simulink model "Teensy41_Cart_Pendulum_SysId"  (R2024b)
settings: Solver=FixedStepAuto  StartTime=0.0  StopTime=18  RelTol=1e-3  EnableMultiTasking=on
InitFcn:
  | run('Teensy41_system_init.m');
StopFcn:
  | run('Teensy41_to_save_data.m');
values from neighbouring files (symbols this model uses):
  Hz_den = Hz.denominator{1}    [Teensy41_system_init.m]
  Hz_num = Hz.numerator{1}    [Teensy41_system_init.m]
  ts = time(2)    [CartPend_SysId.m]    (also in Teensy41_system_init.m = 0.0025)
undefined symbols (not defined in the file or in its folder): dspblkCoreblockFVToolHelper, gcbh
libraries: arduinolib x9, simulink x2, simulink_extras x1
settings Model: SimulationMode=external  ExtModeTrigDuration=2  Creator=ricardoaguilera  LastModifiedBy=ricardoaguilera
settings SolverCC: AutoInsertRateTranBlk=on
settings OptimizationCC: EnhancedBackFolding=on  PassReuseOutputArgsAs=Individual arguments  ZeroExternalMemoryAtStartup=off  ZeroInternalMemoryAtStartup=off  MaxStackSize=64  OptimizeBlockOrder=speed  DifferentSizesBufferReuse=on  OptimizationCustomize=off  EfficientTunableParamExpr=on
settings DebuggingCC: ParameterTunabilityLossMsg=error
settings HardwareCC: ProdBitPerPointer=32  ProdBitPerSizeT=32  ProdBitPerPtrDiffT=32  ProdLargestAtomicInteger=Long  ProdLargestAtomicFloat=Double  ProdWordSize=32  ProdHWDeviceType=ARM Compatible->ARM Cortex
settings SFSimCC: MATLABDynamicMemAlloc=off
settings RTWCC: Description=Embedded Coder  SystemTargetFile=ert.tlc  HardwareBoard=Teensy 4.1 (Arduino Compatible)  TemplateMakefile=ert_default_tmf  Toolchain=Arduino ARM M7  BuildConfiguration=Faster Runs
settings CodeAppCC: ForceParamTrailComments=on  IgnoreCustomStorageClasses=off  OperatorAnnotations=on  SimulinkDataObjDesc=on  SFDataObjDesc=on  InsertBlockDesc=on
settings ERTTargetCC: SupportContinuousTime=on  SupportVariableSizeSignals=on  ExtModeTransport=3  ExtModeStaticAlloc=on  ExtModeAutomaticAllocSize=off  ExtModeStaticAllocSize=65536  ExtModeMexFile=ext_xcp  ExtModeIntrfLevel=Level2 - Open  InlinedParameterPlacement=Hierarchical

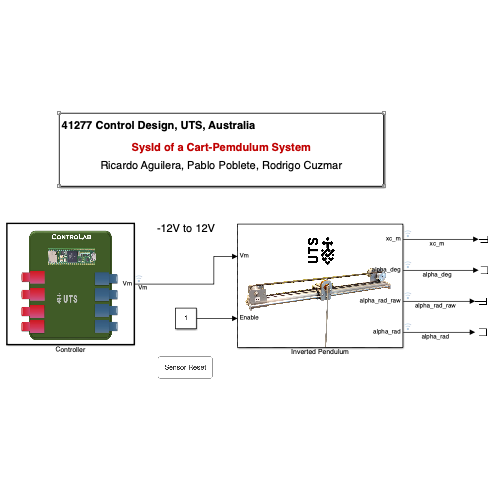
[thumbnail: Simulink's stored preview of the top-level diagram]
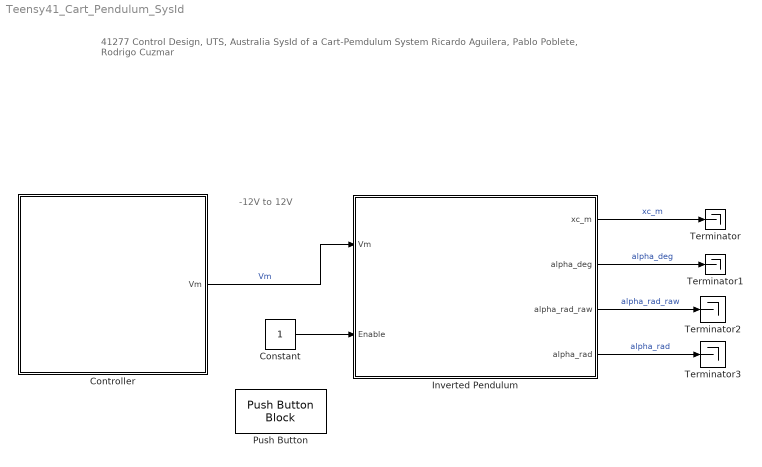
== system Teensy41_Cart_Pendulum_SysId ==
  note: 41277 Control Design, UTS, Australia
      |
      | SysId of a Cart-Pemdulum System
      |
      | Ricardo Aguilera, Pablo Poblete, Rodrigo Cuzmar
  note: -12V to 12V
  Constant : Constant
  Controller : Subsystem  TreatAsAtomicUnit=on
      mask Display: image('Board.png');
  Inverted Pendulum : Subsystem
      mask Display: image('bitmap.png');
  Push Button : PushButtonBlock  ButtonText=Sensor Reset  OffValue=0.000000
  Terminator{,1..3} (4 alike) : Terminator
  wires:
  Inverted Pendulum/1(xc_m) -> Terminator/1  "xc_m"
  Controller/1(Vm) -> Inverted Pendulum/1(Vm)  "Vm"
  Constant/1 -> Inverted Pendulum/2(Enable)
  Inverted Pendulum/4(alpha_rad) -> Terminator3/1  "alpha_rad"
  Inverted Pendulum/3(alpha_rad_raw) -> Terminator2/1  "alpha_rad_raw"
  Inverted Pendulum/2(alpha_deg) -> Terminator1/1  "alpha_deg"

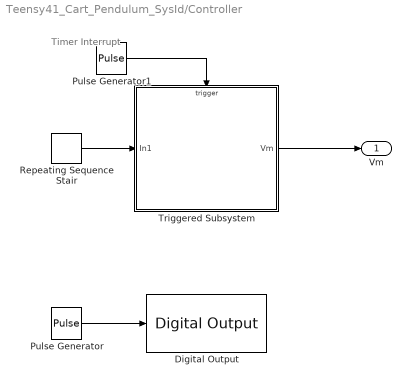
== system Teensy41_Cart_Pendulum_SysId/Controller ==
  note: Timer
      | Interrupt
  Digital Output : arduinolib/Digital Output  pinNumber=13  Direction=output  blockPlatform=arduino
      settings: SourceProductName=Common
  Pulse Generator : DiscretePulseGenerator  PulseType=Time based  Period=4  PulseWidth=50
  Pulse Generator1 : DiscretePulseGenerator  PulseType=Time based  Period=ts  PulseWidth=50
  Repeating Sequence Stair : simulink/Sources/Repeating Sequence Stair  OutValues=6*[0 1 0 0 0 0 0 0 0 -1 0 0 0 0 0 0 0].'  tsamp=1  OutMin=[]  OutMax=[]  OutDataTypeStr=double  OutputDataTypeScalingMode=double  OutDataType=fixdt(0,8)  ConRadixGroup=Best Precision: Vector-wise  OutScaling=2^-12
  Triggered Subsystem : Subsystem  TreatAsAtomicUnit=on
  Vm : Outport
  wires:
  Pulse Generator/1 -> Digital Output/1
  Triggered Subsystem/1(Vm) -> Vm/1
  Pulse Generator1/1 -> Triggered Subsystem/Trigger
  Repeating Sequence Stair/1 -> Triggered Subsystem/1(In1)

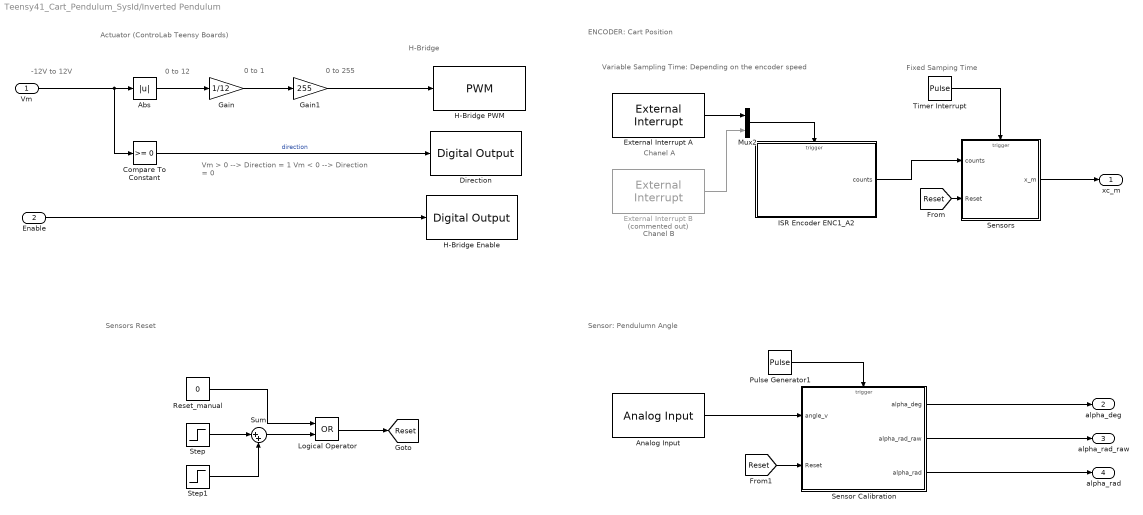
== system Teensy41_Cart_Pendulum_SysId/Inverted Pendulum ==
  note: Fixed Samping Time
  note: H-Bridge
  note: Variable Sampling Time: Depending on the encoder speed
  note: Chanel B
  note: 0 to 1
  note: Sensors Reset
  note: 0 to 12
  note: Chanel A
  note: ENCODER: Cart Position
  note: -12V to 12V
  note: 0 to 255
  note: Vm > 0 --> Direction = 1
      | Vm < 0 --> Direction = 0
  note: Sensor: Pendulumn Angle
  note: Actuator (ControLab Teensy Boards)
  Vm : Inport
  Enable : Inport  Port=2
  Abs : Abs  SaturateOnIntegerOverflow=off
  Analog Input : arduinolib/Analog Input  pinNumber=0  ReadResultsOnly=off  ConversionTriggerSource=Software  ExternalTriggerType=uint32( 0 )  OutputDataType=uint16  EnableConversionCompleteNotify=off  EnableOuputStatus=off  SampleTime=ts  blockPlatform=arduino
      settings: SourceProductName=Common
  Compare To Constant : simulink/Logic and Bit Operations/Compare To Constant  relop=>=  const=0  OutDataTypeStr=boolean
  Direction : arduinolib/Digital Output  pinNumber=8  Direction=output  blockPlatform=arduino
      settings: SourceProductName=Common
  "External Interrupt A " : arduinolib/External Interrupt  Pin=29  PullUp=off  Mode=CHANGE  InterruptSimulationInput=off
      settings: SourceProductName=Common
  External Interrupt B : arduinolib/External Interrupt  Commented=on  Pin=5  PullUp=off  Mode=CHANGE  InterruptSimulationInput=off
      settings: SourceProductName=Common
  Gain : Gain  Gain=1/12
  Gain1 : Gain  Gain=255
  H-Bridge Enable : arduinolib/Digital Output  pinNumber=9  Direction=output  blockPlatform=arduino
      settings: SourceProductName=Common
  H-Bridge PWM : arduinolib/PWM  pinNumber=3  frequencyType=Specify  desiredFrequency=10000  achievableFrequency=10000
      settings: SourceProductName=Common
  ISR Encoder ENC1_A2 : Subsystem  TreatAsAtomicUnit=on
  Logical Operator : Logic  Operator=OR  AllPortsSameDT=off  OutDataTypeStr=boolean
  Mux2 : Mux  Inputs=2
  Pulse Generator1 : DiscretePulseGenerator  PulseType=Time based  Period=ts  PulseWidth=50
  Reset_manual : Constant  Value=0  SampleTime=-1
  Sensor Calibration : Subsystem
  Sensors : Subsystem
  Step : Step  Time=ts
  Step1 : Step  Time=2*ts  After=-1
  Sum : Sum  Inputs=|++
  Timer Interrupt : DiscretePulseGenerator  PulseType=Time based  Period=ts  PulseWidth=50
  xc_m : Outport
  alpha_deg : Outport  Port=2
  alpha_rad_raw : Outport  Port=3
  alpha_rad : Outport  Port=4
  tag scope: Reset=global
  wires:
  ISR Encoder ENC1_A2/1(counts) -> Sensors/1(counts)
  Timer Interrupt/1 -> Sensors/Trigger
  Mux2/1 -> ISR Encoder ENC1_A2/Trigger
  Vm/1 -> Compare To Constant/1, Abs/1
  Compare To Constant/1 -> Direction/1  "direction"
  Abs/1 -> Gain/1
  External Interrupt B/1 -> Mux2/2
  Gain/1 -> Gain1/1
  Enable/1 -> H-Bridge Enable/1
  Gain1/1 -> H-Bridge PWM/1
  "External Interrupt A "/1 -> Mux2/1
  Analog Input/1 -> Sensor Calibration/1(angle_v)
  Sensor Calibration/3(alpha_rad) -> alpha_rad/1
  Pulse Generator1/1 -> Sensor Calibration/Trigger
  [Reset] -> Sensors/2(Reset)
  Sensors/1(x_m) -> xc_m/1
  [Reset] -> Sensor Calibration/2(Reset)
  Logical Operator/1 -> [Reset]
  Step/1 -> Sum/1
  Step1/1 -> Sum/2
  Sum/1 -> Logical Operator/2
  Reset_manual/1 -> Logical Operator/1
  Sensor Calibration/2(alpha_rad_raw) -> alpha_rad_raw/1
  Sensor Calibration/1(alpha_deg) -> alpha_deg/1

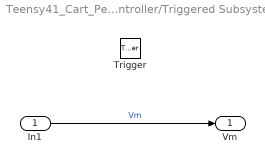
== system Teensy41_Cart_Pendulum_SysId/Controller/Triggered Subsystem ==
  In1 : Inport
  Trigger : TriggerPort  VariantControl=(inherit)
  Vm : Outport
  wires:
  In1/1 -> Vm/1  "Vm"

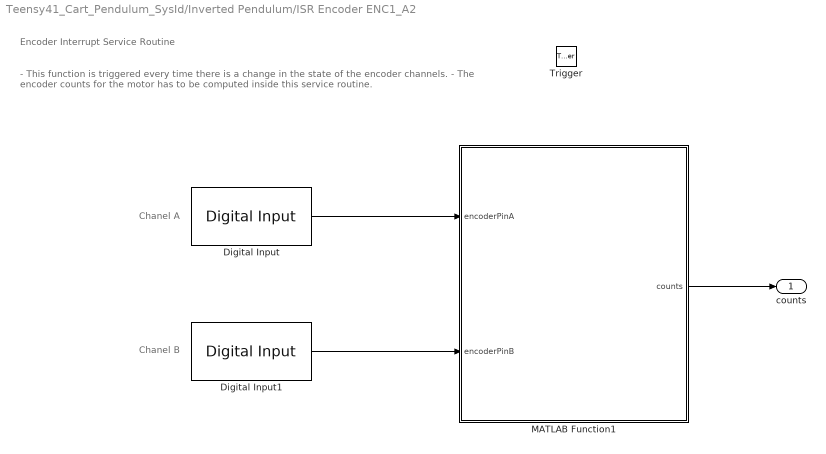
== system Teensy41_Cart_Pendulum_SysId/Inverted Pendulum/ISR Encoder ENC1_A2 ==
  note: - This function is triggered every time there is a change in the state of the encoder channels.
      | - The encoder counts for the motor has to be computed inside this service routine.
  note: Encoder Interrupt Service Routine
  note: Chanel A
  note: Chanel B
  Trigger : TriggerPort  TriggerType=function-call  VariantControl=(inherit)
  Digital Input : arduinolib/Digital Input  pinNumber=30  mode=Default  Direction=input  SampleTime=-1  blockPlatform=arduino
      settings: SourceProductName=Common
  Digital Input1 : arduinolib/Digital Input  pinNumber=31  mode=Default  Direction=input  SampleTime=-1  blockPlatform=arduino
      settings: SourceProductName=Common
  MATLAB Function1 : MATLAB Function  TreatAsAtomicUnit=on
  counts : Outport
  wires:
  MATLAB Function1/1(counts) -> counts/1
  Digital Input/1 -> MATLAB Function1/1(encoderPinA)
  Digital Input1/1 -> MATLAB Function1/2(encoderPinB)

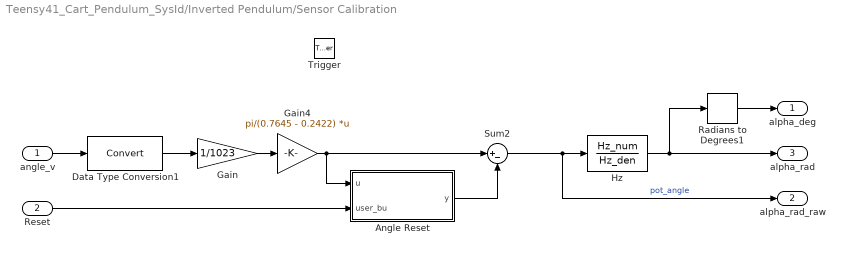
== system Teensy41_Cart_Pendulum_SysId/Inverted Pendulum/Sensor Calibration ==
  angle_v : Inport
  Reset : Inport  Port=2
  Trigger : TriggerPort  VariantControl=(inherit)  PortDimensions=1
  Angle Reset : MATLAB Function  TreatAsAtomicUnit=on
  Data Type Conversion1 : DataTypeConversion  SaturateOnIntegerOverflow=off  RndMeth=Floor
  Gain : Gain  Gain=1/1023
  Gain4 : Gain  Gain=pi/(0.7645 - 0.2422)  Multiplication=Matrix(K*u)
  Hz : DiscreteTransferFcn  LoadFcn=dspblkCoreblockFVToolHelper(gcbh,'load');  Numerator=Hz_num  Denominator=Hz_den
      settings: CopyFcn=dspblkCoreblockFVToolHelper(gcbh,'copy');  DeleteFcn=dspblkCoreblockFVToolHelper(gcbh,'close');  ModelCloseFcn=dspblkCoreblockFVToolHelper(gcbh,'close');  PreSaveFcn=dspblkCoreblockFVToolHelper(gcbh,'presave');  PostSaveFcn=dspblkCoreblockFVToolHelper(gcbh,'postsave');  CloseFcn=dspblkCoreblockFVToolHelper(gcbh,'close');
  Radians to Degrees1 : simulink_extras/Transformations/Radians to Degrees
  Sum2 : Sum  Inputs=|+-
  alpha_deg : Outport
  alpha_rad_raw : Outport  Port=2
  alpha_rad : Outport  Port=3
  wires:
  Angle Reset/1(y) -> Sum2/2
  Sum2/1 -> alpha_rad_raw/1, Hz/1  "pot_angle"
  Gain4/1 -> Angle Reset/1(u), Sum2/1
  Reset/1 -> Angle Reset/2(user_bu)
  angle_v/1 -> Data Type Conversion1/1
  Gain/1 -> Gain4/1
  Data Type Conversion1/1 -> Gain/1
  Hz/1 -> Radians to Degrees1/1, alpha_rad/1
  Radians to Degrees1/1 -> alpha_deg/1

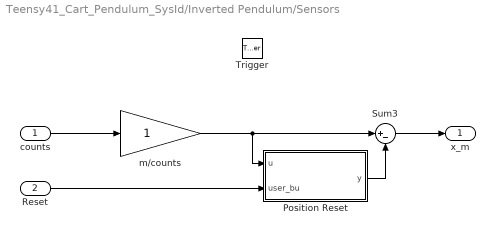
== system Teensy41_Cart_Pendulum_SysId/Inverted Pendulum/Sensors ==
  counts : Inport
  Reset : Inport  Port=2
  Trigger : TriggerPort  VariantControl=(inherit)  PortDimensions=1
  Position Reset : MATLAB Function  TreatAsAtomicUnit=on
  Sum3 : Sum  Inputs=|+-
  m/counts : Gain
  x_m : Outport
  wires:
  Sum3/1 -> x_m/1
  Reset/1 -> Position Reset/2(user_bu)
  m/counts/1 -> Position Reset/1(u), Sum3/1
  Position Reset/1(y) -> Sum3/2
  counts/1 -> m/counts/1

== matlab function Teensy41_Cart_Pendulum_SysId/Inverted Pendulum/Sensors/Position Reset ==
  data: u input; y output; user_bu input
function y = fcn(u, user_bu)

persistent offset u_vec

if isempty(offset)
    offset = 0;
    u_vec = zeros(20,1);
end

if(user_bu == 1)
    u_vec = [u ; u_vec(1:end-1)];
    offset = mean(u);
end

y = offset;

end

== matlab function Teensy41_Cart_Pendulum_SysId/Inverted Pendulum/Sensor Calibration/Angle Reset ==
  data: u input; y output size=1; user_bu input
function y = fcn(u, user_bu)

persistent offset u_vec

if isempty(offset)
    offset = 0;
    u_vec = zeros(20,1);
end

if(user_bu == 1)
    u_vec = [u ; u_vec(1:end-1)];
    offset = mean(u);
end

y = offset;

end

== matlab function Teensy41_Cart_Pendulum_SysId/Inverted Pendulum/ISR Encoder ENC1_A2/MATLAB Function1 ==
  data: counts output; encoderPinA input; encoderPinB input
function counts = computeEncoderPosition(encoderPinA, encoderPinB)
% This function determines the motor position based on the latest 
% state update for the encoder digital inputs. 

%% Persistent variables to store previous states and position
persistent lastPosition

% Initialize persistent variables on the first run
if isempty(lastPosition)

    lastPosition = 0;
end


%% Determine direction and update position
if (encoderPinA == encoderPinB)
    % Direction is forward
    lastPosition = lastPosition + 1;
else
    % Direction is backward
    lastPosition = lastPosition - 1;
end

%% Output the current position
counts = lastPosition;
